simulink model "NonlinearEKF_Kim"  (R2019b)
settings: Solver=FixedStepAuto  StartTime=0.0  StopTime=10.0  FixedStep=0.01  RelTol=1e-3
settings Model: Creator=김태욱  LastModifiedBy=김태욱

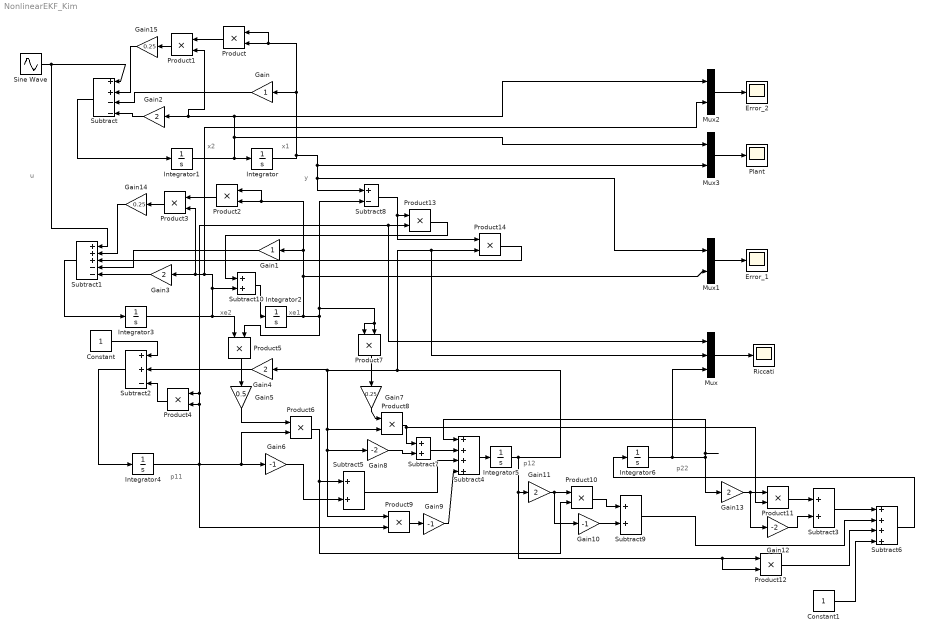
== system NonlinearEKF_Kim ==
  note: u
  note: y
  note: p22
  note: p12
  note: xe2
  note: p11
  note: x2
  note: x1
  note: xe1
  Constant : Constant
  Constant1 : Constant
  Error_1 : Scope
  Error_2 : Scope
  Gain : Gain
  Gain1 : Gain
  Gain10 : Gain  Gain=-1
  Gain{2..4,11,13} (5 alike) : Gain  Gain=2
  Gain12 : Gain  Gain=-2
  Gain14 : Gain  Gain=0.25
  Gain15 : Gain  Gain=0.25
  Gain5 : Gain  Gain=0.5
  Gain6 : Gain  Gain=-1
  Gain7 : Gain  Gain=0.25
  Gain8 : Gain  Gain=-2
  Gain9 : Gain  Gain=-1
  Integrator : Integrator  InitialCondition=1
  Integrator1 : Integrator  InitialCondition=-1
  Integrator2 : Integrator
  Integrator3 : Integrator
  Integrator4 : Integrator  InitialCondition=1
  Integrator5 : Integrator
  Integrator6 : Integrator  InitialCondition=1
  Mux : Mux  Inputs=3
  Mux1 : Mux  Inputs=2
  Mux2 : Mux  Inputs=2
  Mux3 : Mux  Inputs=2
  Plant : Scope
  Product{,1..14} (15 alike) : Product
  Riccati : Scope
  Sine Wave : Sin  Amplitude=0.25  Frequency=2  SampleTime=0
  Subtract : Sum  Inputs=++--
  Subtract1 : Sum  Inputs=+++--
  Subtract{3,5,7,9..10} (5 alike) : Sum
  Subtract2 : Sum  Inputs=++-
  Subtract4 : Sum  Inputs=++++
  Subtract6 : Sum  Inputs=++++
  Subtract8 : Sum  Inputs=+-
  wires:
  Integrator/1 -> Mux3/2, Mux1/1, Subtract8/1, Gain/1, Product/1, Product/2
  Integrator1/1 -> Mux3/1, Mux2/1, Gain2/1, Product1/2, Integrator/1
  Product/1 -> Product1/1
  Gain2/1 -> Subtract/4
  Gain/1 -> Subtract/3
  Sine Wave/1 -> Subtract/1, Subtract1/1
  Subtract/1 -> Integrator1/1
  Subtract1/1 -> Integrator3/1
  Product2/1 -> Product3/1
  Integrator4/1 -> Mux/1, Product13/2, Product4/1, Product4/2, Product9/2, Product6/2, Gain6/1
  Product4/1 -> Subtract2/3
  Gain4/1 -> Subtract2/2
  Constant/1 -> Subtract2/1
  Subtract2/1 -> Integrator4/1
  Product5/1 -> Gain5/1
  Gain5/1 -> Product6/1
  Product7/1 -> Gain7/1
  Gain7/1 -> Product8/1
  Integrator6/1 -> Mux/3, Subtract4/1, Gain13/1
  Subtract4/1 -> Integrator5/1
  Product6/1 -> Product10/2, Subtract5/1
  Gain6/1 -> Subtract5/2
  Gain8/1 -> Subtract7/2
  Subtract7/1 -> Subtract4/2
  Product9/1 -> Gain9/1
  Subtract5/1 -> Subtract4/3
  Gain9/1 -> Subtract4/4
  Gain11/1 -> Gain10/1, Product10/1
  Product10/1 -> Subtract9/1
  Gain10/1 -> Subtract9/2
  Product8/1 -> Product11/2, Subtract7/1
  Gain13/1 -> Gain12/1, Product11/1
  Product11/1 -> Subtract3/1
  Gain12/1 -> Subtract3/2
  Subtract3/1 -> Subtract6/1
  Constant1/1 -> Subtract6/4
  Subtract9/1 -> Subtract6/2
  Product12/1 -> Subtract6/3
  Subtract6/1 -> Integrator6/1
  Integrator2/1 -> Product2/2, Product2/1, Gain1/1, Mux1/2, Product7/1, Product7/2, Subtract8/2, Product5/2
  Subtract8/1 -> Product14/1, Product13/1
  Product13/1 -> Subtract10/1
  Integrator3/1 -> Product5/1, Mux2/2, Product3/2, Gain3/1, Subtract10/2
  Subtract10/1 -> Integrator2/1
  Product3/1 -> Gain14/1
  Gain14/1 -> Subtract1/2
  Gain3/1 -> Subtract1/5
  Gain1/1 -> Subtract1/4
  Product14/1 -> Subtract1/3
  Mux/1 -> Riccati/1
  Mux1/1 -> Error_1/1
  Mux2/1 -> Error_2/1
  Mux3/1 -> Plant/1
  Integrator5/1 -> Gain4/1, Product8/2, Gain8/1, Product9/1, Mux/2, Product14/2, Gain11/1, Product12/2, Product12/1
  Product1/1 -> Gain15/1
  Gain15/1 -> Subtract/2
